simulink model "DC-Motor_simulation"  (R2020a)
settings: Solver=VariableStepAuto  StartTime=0.0  StopTime=10.0  RelTol=1e-3
libraries: arduinolib x2
settings Model: Creator=junio  LastModifiedBy=junio

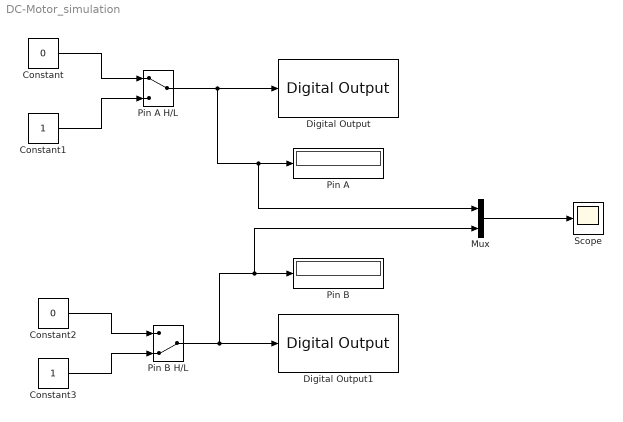
== system DC-Motor_simulation ==
  Constant : Constant  Value=0
  Constant1 : Constant
  Constant2 : Constant  Value=0
  Constant3 : Constant
  Digital Output : arduinolib/Digital Output  pinNumber=9  Direction=output  blockPlatform=arduino
  Digital Output1 : arduinolib/Digital Output  pinNumber=10  Direction=output  blockPlatform=arduino
  Mux : Mux  Inputs=2
  Pin A : Display
  Pin A H/L : ManualSwitch
  Pin B : Display
  Pin B H/L : ManualSwitch  CurrentSetting=0
  Scope : Scope
  wires:
  Pin A H/L/1 -> Digital Output/1, Mux/1, Pin A/1
  Pin B H/L/1 -> Digital Output1/1, Pin B/1, Mux/2
  Constant2/1 -> Pin B H/L/1
  Constant3/1 -> Pin B H/L/2
  Constant/1 -> Pin A H/L/1
  Constant1/1 -> Pin A H/L/2
  Mux/1 -> Scope/1
